simulink model "sampleModel6"  (R2021b)
settings: Solver=VariableStepAuto  StartTime=0.0  StopTime=10.0  RelTol=1e-3
undefined symbols (not defined in the file or in its folder): DiscIntNeverNeededParam
libraries: simulink x11, slpidlib x1
settings Model: Creator=user  LastModifiedBy=user

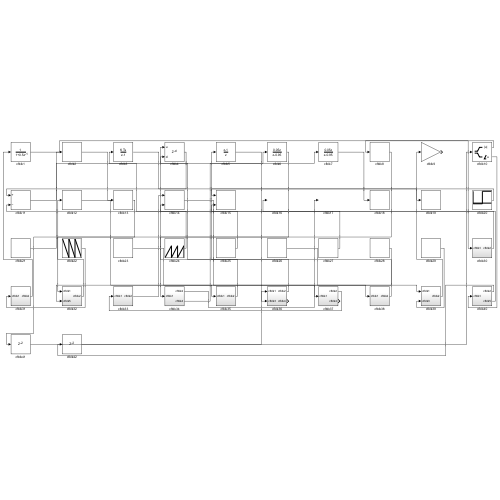
[thumbnail: Simulink's stored preview of the top-level diagram]
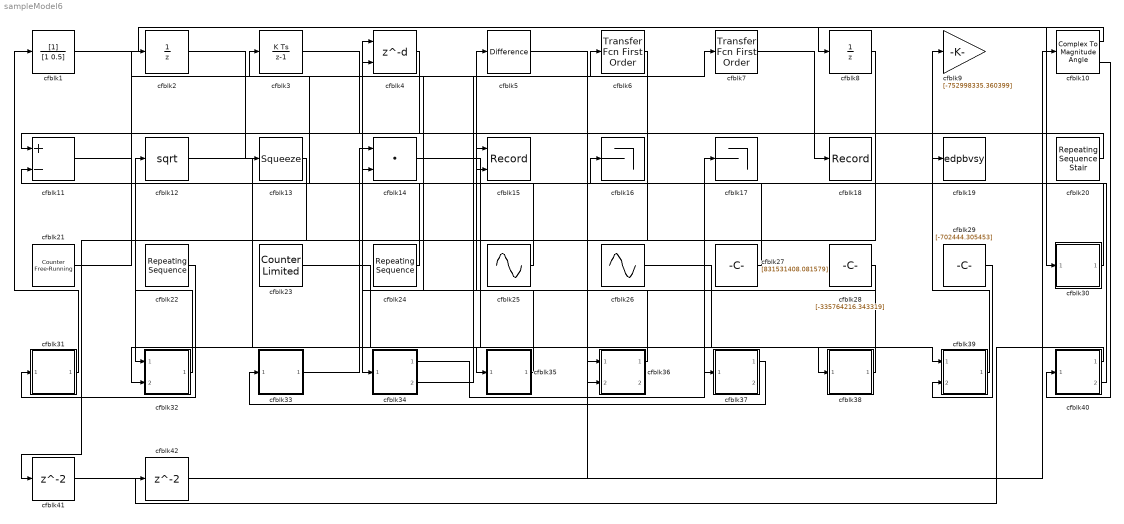
== system sampleModel6 ==
  cfblk1 : DiscreteFilter  SampleTime=1
  cfblk10 : ComplexToMagnitudeAngle
  cfblk11 : Sum  Inputs=+-
  cfblk12 : Sqrt  SaturateOnIntegerOverflow=on
  cfblk13 : Squeeze
  cfblk14 : DotProduct  InputSameDT=on  OutDataTypeStr=Inherit: Inherit via internal rule
  cfblk15 : Record  FileSettingsInternal="{\"entries\":[{\"content\":{\"excelSettings\":{\"content\":{},\"type\":\"Streamout.ExcelSettings\"}},\"type\":\"Streamout.FileSettingStorage\",\"uuid\":\"078a0047-3eb5-4cfb-884a-48a50617e5a1\"}],\"packageUris\":[\"http://schema.mathworks.com/mf0/streamout_blocks/R2020a\"],\"version\":\"1.0\"}"  Layout=[1 1]  SignalsInternal="{\"entries\":[{\"content\":{\"signals\":[{\"content\":{\"blockPath\":[\"sampleModel6/cfblk15\"],\"channel\":[],\"dimensions\":[1],\"domain\":\"sampleModel6/cfblk15\",\"lineColor\":\"#a2142f\",\"plots\":[1],\"port\":1,\"sid\":[\"\"],\"signalID\":237,\"signalName\":\"cfblk20\"},\"type\":\"RecordBlkView.Signal\",\"uuid\":\"e2950a3c-6211-4e69-b9c2-83c3ff1a6d9b\"},{\"content\":{\"blockPath\":[\"sampleModel6/cfblk15\"],\"channel\":[],\"dimensions\":[1],\"domain\":\"sampleModel6/cfblk15\",\"lineColor\":\"#139fff\",\"plots\":[1],\"port\":2,\"sid\":[\"\"],\"signalID\":241,\"signalName\":\"cfblk30\"},\"type\":\"RecordBlkView.Signal\",\"uuid\":\"a62bb186-0eaa-4d5d-9c06-4d8813e13515\"}]},\"type\":\"RecordBlkView.InputSignals\",\"uuid\":\"a1dddcb4-b3bf-44b7-b4b8-68e776bbfcf3\"}],\"packageUris\":[\"http://schema.mathworks.com/mf0/streamout_blocks/R2020a\"],\"version\":\"1.0\"}"  VisualizationBindings="{\"xyplotplugin\":{\"info\":[{\"series\":[{\"bindingParametersList\":[{\"parameter\":\"X-Axis\",\"signalID\":237,\"signalName\":\"cfblk20\"},{\"parameter\":\"Y-Axis\",\"signalID\":241,\"signalName\":\"cfblk30\"}],\"seriesID\":36112}],\"subplotID\":1}]}}"  CompatibilityTag=XY
  cfblk16 : Terminator
  cfblk17 : Terminator
  cfblk18 : Record  FileSettingsInternal="{\"entries\":[{\"content\":{\"excelSettings\":{\"content\":{},\"type\":\"Streamout.ExcelSettings\"}},\"type\":\"Streamout.FileSettingStorage\",\"uuid\":\"ff4303cd-4097-4d51-a6e8-73b3556a0e5d\"}],\"packageUris\":[\"http://schema.mathworks.com/mf0/streamout_blocks/R2020a\"],\"version\":\"1.0\"}"  SignalsInternal="{\"entries\":[{\"content\":{\"signals\":[{\"content\":{\"blockPath\":[\"sampleModel6/cfblk18\"],\"channel\":[],\"dimensions\":[1],\"domain\":\"sampleModel6/cfblk18\",\"lineColor\":\"#d95319\",\"plots\":[1],\"port\":1,\"sid\":[\"\"],\"signalID\":233,\"signalName\":\"cfblk7\"},\"type\":\"RecordBlkView.Signal\",\"uuid\":\"350a4dd6-4f43-4d64-a145-38d7b0e854d1\"}]},\"type\":\"RecordBlkView.InputSignals\",\"uuid\":\"cfb04e90-a252-4558-a39a-d3efc5ac2aac\"}],\"packageUris\":[\"http://schema.mathworks.com/mf0/streamout_blocks/R2020a\"],\"version\":\"1.0\"}"  VisualizationBindings="{\"sparklinesplugin\":{\"info\":[{\"bindingParametersList\":[],\"subplotID\":1}]}}"
  cfblk19 : ToWorkspace  VariableName=edpbvsy  SaveFormat=Timeseries  SampleTime=-1
  cfblk2 : UnitDelay  HasFrameUpgradeWarning=on
  cfblk20 : simulink/Sources/Repeating Sequence Stair  OutValues=[-14722803.076438, 309765796.899337]  tsamp=-1  OutMin=[]  OutMax=[]  OutDataTypeStr=double  OutputDataTypeScalingMode=double  OutDataType=fixdt(0,8)  ConRadixGroup=Best Precision: Vector-wise  OutScaling=2^-12
  cfblk21 : simulink/Sources/Counter Free-Running  NumBits=[53.000000]  tsamp=-1
  cfblk22 : simulink/Sources/Repeating Sequence  rep_seq_t=[0 2]  rep_seq_y=[77051148.938042, -435589670.883555]
  cfblk23 : simulink/Sources/Counter Limited  uplimit=[975.000000]  tsamp=-1
  cfblk24 : simulink/Sources/Repeating Sequence  rep_seq_t=[0 2]  rep_seq_y=[-927148968.949040, -347510853.879375]
  cfblk25 : Sin  Amplitude=[946027247.785641]  Bias=[-269934749.388505]  SampleTime=0
  cfblk26 : Sin  Amplitude=[-381700762.208165]  Bias=[-758175230.838743]  SampleTime=0
  cfblk27 : Constant  Value=[831531408.081579]  SampleTime=1
  cfblk28 : Constant  Value=[-335764216.343319]  SampleTime=1
  cfblk29 : Constant  Value=[-702444.305453]  SampleTime=1
  cfblk3 : DiscreteIntegrator  ICPrevOutput=DiscIntNeverNeededParam  ICPrevScaledInput=DiscIntNeverNeededParam
  cfblk30 : Subsystem
  cfblk31 : Subsystem
  cfblk32 : Subsystem
  cfblk33 : Subsystem
  cfblk34 : Subsystem
  cfblk35 : Subsystem
  cfblk36 : Subsystem
  cfblk37 : Subsystem
  cfblk38 : Subsystem
  cfblk39 : Subsystem
  cfblk4 : Delay  DelayLengthSource=Input port  SampleTime=1
      settings: InputPortMap=u0,p1
  cfblk40 : Subsystem
  cfblk41 : Delay  SampleTime=1
  cfblk42 : Delay  SampleTime=1
  cfblk5 : simulink/Discrete/Difference  ICPrevInput=0.0  OutMin=[]  OutMax=[]  OutDataTypeStr=Inherit: Inherit via back propagation  OutDataType=fixdt(1, 16)  OutScaling=2^-10  DoSatur=off
  cfblk6 : simulink/Discrete/Transfer Fcn First Order  PoleZ=0.95  ICPrevOutput=0.0  DoSatur=off
  cfblk7 : simulink/Discrete/Transfer Fcn First Order  PoleZ=0.95  ICPrevOutput=0.0  DoSatur=off
  cfblk8 : UnitDelay  HasFrameUpgradeWarning=on
  cfblk9 : Gain  Gain=[-752998335.360399]
  wires:
  cfblk12/1 -> cfblk35/1(cfblk1)
  cfblk24/1 -> cfblk3/1
  cfblk32/1(cfblk2) -> cfblk12/1
  cfblk34/1(cfblk2) -> cfblk17/1
  cfblk35/1(cfblk2) -> cfblk5/1
  cfblk1/1 -> cfblk30/1(cfblk1)
  cfblk23/1 -> cfblk38/1(cfblk1)
  cfblk27/1 -> cfblk16/1
  cfblk37/1(cfblk2) -> cfblk33/1(cfblk1)
  cfblk4/1 -> cfblk11/1
  cfblk13/1 -> cfblk32/1(cfblk1)
  cfblk14/1 -> cfblk36/2(cfblk3)
  cfblk8/1 -> cfblk34/1(cfblk1)
  cfblk38/1(cfblk2) -> cfblk4/1
  cfblk31/1(cfblk2) -> cfblk1/1
  cfblk22/1 -> cfblk31/1(cfblk1)
  cfblk25/1 -> cfblk11/2
  cfblk11/1 -> cfblk6/1
  cfblk39/1(cfblk2) -> cfblk9/1
  cfblk10/1 -> cfblk8/1
  cfblk33/1(cfblk2) -> cfblk14/1
  cfblk36/1(cfblk2) -> cfblk4/2
  cfblk21/1 -> cfblk2/1
  cfblk34/2(cfblk4) -> cfblk7/1
  cfblk5/1 -> cfblk37/1(cfblk1)
  cfblk28/1 -> cfblk32/2(cfblk5)
  cfblk26/1 -> cfblk39/1(cfblk1)
  cfblk10/2 -> cfblk40/1(cfblk1)
  cfblk20/1 -> cfblk15/1
  cfblk40/2(cfblk5) -> cfblk14/2
  cfblk7/1 -> cfblk18/1
  cfblk30/1(cfblk2) -> cfblk15/2
  cfblk3/1 -> cfblk19/1
  cfblk29/1 -> cfblk39/2(cfblk3)
  cfblk2/1 -> cfblk13/1
  cfblk6/1 -> cfblk41/1
  cfblk41/1 -> cfblk36/1(cfblk1)
  cfblk40/1(cfblk2) -> cfblk42/1
  cfblk42/1 -> cfblk10/1

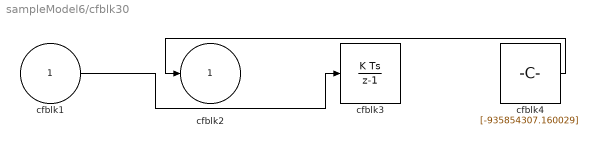
== system sampleModel6/cfblk30 ==
  cfblk1 : Inport
  cfblk3 : DiscreteIntegrator  ICPrevOutput=DiscIntNeverNeededParam  ICPrevScaledInput=DiscIntNeverNeededParam
  cfblk4 : Constant  Value=[-935854307.160029]  SampleTime=1
  cfblk2 : Outport
  wires:
  cfblk4/1 -> cfblk2/1
  cfblk1/1 -> cfblk3/1

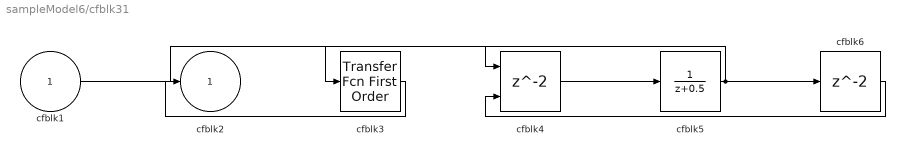
== system sampleModel6/cfblk31 ==
  cfblk1 : Inport
  cfblk3 : simulink/Discrete/Transfer Fcn First Order  PoleZ=0.95  ICPrevOutput=0.0  DoSatur=off
  cfblk4 : Delay  ShowEnablePort=on  SampleTime=1
      settings: InputPortMap=u0,e6
  cfblk5 : DiscreteTransferFcn  SampleTime=1
  cfblk6 : Delay  SampleTime=1
  cfblk2 : Outport
  wires:
  cfblk1/1 -> cfblk4/1
  cfblk3/1 -> cfblk2/1
  cfblk4/1 -> cfblk5/1
  cfblk5/1 -> cfblk3/1, cfblk6/1
  cfblk6/1 -> cfblk4/2

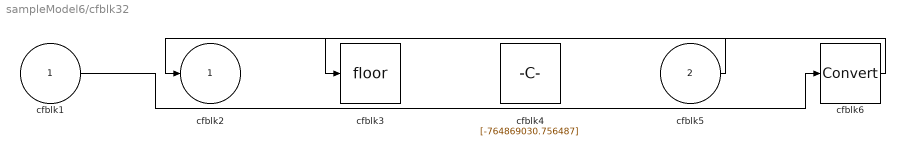
== system sampleModel6/cfblk32 ==
  cfblk1 : Inport
  cfblk5 : Inport  Port=2
  cfblk3 : Rounding
  cfblk4 : Constant  Value=[-764869030.756487]  SampleTime=1
  cfblk6 : DataTypeConversion
  cfblk2 : Outport
  wires:
  cfblk5/1 -> cfblk2/1
  cfblk1/1 -> cfblk6/1
  cfblk6/1 -> cfblk3/1

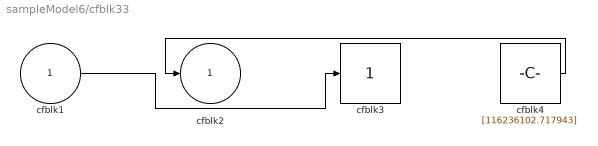
== system sampleModel6/cfblk33 ==
  cfblk1 : Inport
  cfblk3 : simulink/Math Operations/Slider Gain  gain=1  low=0  high=2
  cfblk4 : Constant  Value=[116236102.717943]  SampleTime=1
  cfblk2 : Outport
  wires:
  cfblk4/1 -> cfblk2/1
  cfblk1/1 -> cfblk3/1

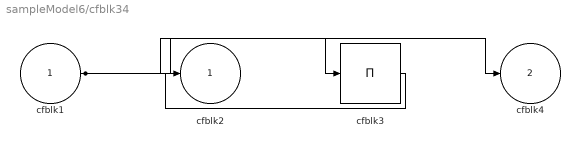
== system sampleModel6/cfblk34 ==
  cfblk1 : Inport
  cfblk3 : Product  Inputs=*
  cfblk2 : Outport
  cfblk4 : Outport  Port=2
  wires:
  cfblk1/1 -> cfblk4/1, cfblk3/1
  cfblk3/1 -> cfblk2/1

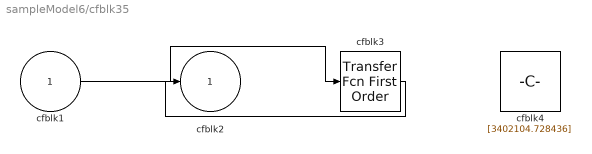
== system sampleModel6/cfblk35 ==
  cfblk1 : Inport
  cfblk3 : simulink/Discrete/Transfer Fcn First Order  PoleZ=0.95  ICPrevOutput=0.0  DoSatur=off
  cfblk4 : Constant  Value=[3402104.728436]  SampleTime=1
  cfblk2 : Outport
  wires:
  cfblk1/1 -> cfblk3/1
  cfblk3/1 -> cfblk2/1

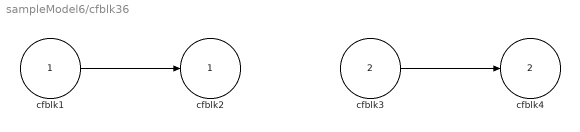
== system sampleModel6/cfblk36 ==
  cfblk1 : Inport
  cfblk3 : Inport  Port=2
  cfblk2 : Outport
  cfblk4 : Outport  Port=2
  wires:
  cfblk1/1 -> cfblk2/1
  cfblk3/1 -> cfblk4/1

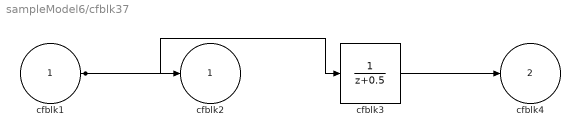
== system sampleModel6/cfblk37 ==
  cfblk1 : Inport
  cfblk3 : DiscreteTransferFcn  SampleTime=1
  cfblk2 : Outport
  cfblk4 : Outport  Port=2
  wires:
  cfblk1/1 -> cfblk2/1, cfblk3/1
  cfblk3/1 -> cfblk4/1

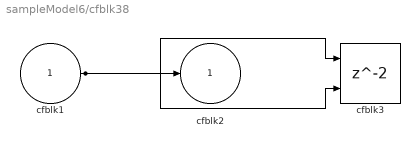
== system sampleModel6/cfblk38 ==
  cfblk1 : Inport
  cfblk3 : Delay  ShowEnablePort=on  SampleTime=1
      settings: InputPortMap=u0,e6
  cfblk2 : Outport
  wires:
  cfblk1/1 -> cfblk2/1, cfblk3/1, cfblk3/2

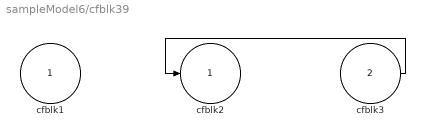
== system sampleModel6/cfblk39 ==
  cfblk1 : Inport
  cfblk3 : Inport  Port=2
  cfblk2 : Outport
  wires:
  cfblk3/1 -> cfblk2/1

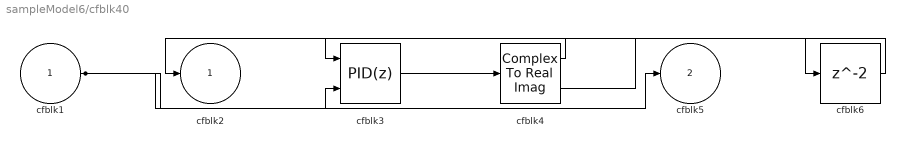
== system sampleModel6/cfblk40 ==
  cfblk1 : Inport
  cfblk3 : slpidlib/PID Controller (2DOF)  Controller=PID  Form=Parallel  TimeDomain=Discrete-time  UseExternalTs=off  SampleTime=1  IntegratorMethod=Forward Euler  FilterMethod=Forward Euler  ControllerParametersSource=internal  P=1  I=1  D=0  UseFilter=on  N=100  b=1  c=1  TunerSelectOption=Transfer Function Based (PID Tuner App)  InitialConditionSource=internal  InitialConditionForIntegrator=0  InitialConditionForFilter=0  DifferentiatorICPrevScaledInput=0  ExternalReset=none  TrackingMode=off  Kt=1  LimitOutput=off  SatLimitsSource=internal  UpperSaturationLimit=inf  LowerSaturationLimit=-inf  LinearizeAsGain=off  AntiWindupMode=none  Kb=1  POutMin=[]  POutMax=[]  IOutMin=[]  IOutMax=[]  DOutMin=[]  DOutMax=[]  NOutMin=[]  NOutMax=[]  bOutMin=[]  bOutMax=[]  cOutMin=[]  cOutMax=[]  SumOutMin=[]  SumOutMax=[]  SaturationOutMin=[]  SaturationOutMax=[]  PParamMin=[]  PParamMax=[]  IParamMin=[]  IParamMax=[]  DParamMin=[]  DParamMax=[]  NParamMin=[]  NParamMax=[]  bParamMin=[]  bParamMax=[]  cParamMin=[]  cParamMax=[]  KbParamMin=[]  KbParamMax=[]  KtParamMin=[]  KtParamMax=[]  KbOutMin=[]  KbOutMax=[]  KtOutMin=[]  KtOutMax=[]  IntegratorOutMin=[]  IntegratorOutMax=[]  FilterOutMin=[]  FilterOutMax=[]  SumI1OutMin=[]  SumI1OutMax=[]  SumI2OutMin=[]  SumI2OutMax=[]  SumI3OutMin=[]  SumI3OutMax=[]  SumI4OutMin=[]  SumI4OutMax=[]  SumDOutMin=[]  SumDOutMax=[]  Sum1OutMin=[]  Sum1OutMax=[]  Sum2OutMin=[]  Sum2OutMax=[]  Sum3OutMin=[]  Sum3OutMax=[]  DifferentiatorOutMin=[]  DifferentiatorOutMax=[]  FilterDiffOutCoefMin=[]  FilterDiffOutCoefMax=[]  ReciprocalOutMin=[]  ReciprocalOutMax=[]  SumDenOutMin=[]  SumDenOutMax=[]  SumNumOutMin=[]  SumNumOutMax=[]  DivideOutMin=[]  DivideOutMax=[]  UdiffTsProdOutMin=[]  UdiffTsProdOutMax=[]  NTsProdOutMin=[]  NTsProdOutMax=[]  UintegralTsProdOutMin=[]  UintegralTsProdOutMax=[]  UngainTsProdOutMin=[]  UngainTsProdOutMax=[]  IntegratorContinuousStateAttributes=''  IntegratorStateMustResolveToSignalObject=off  IntegratorRTWStateStorageClass=Auto  FilterContinuousStateAttributes=''  FilterStateMustResolveToSignalObject=off  FilterRTWStateStorageClass=Auto  ParallelPVariant=InternalParameters  IdealPVariant=Disabled  IVariant=InternalParameters  DVariant=InternalParameters  bVariant=InternalParameters  cVariant=InternalParameters  IntegratorVariant=Discrete  SatVariant=Disabled  AWVariant=Passthrough  PCopyVariant=Disabled  TRVariant=Disabled  FdbkBlocksVariant=Forward  IdealPFdbkVariant=Disabled  SatFdbkVariant=Disabled  DerivativeFilterVariant=ForwardEulerFilter  NVariant=InternalParameters  NCopyVariant=Disabled  FilterICVariant=InternalICsFilter  IntegratorICVariant=InternalICs  ExternalResetVariant=Disabled  TRSumVariant=Passthrough  SumFdbkVariant=Disabled  SumVariant=Sum_PID  TsampFilterVariant=InternalTs  TsampNgainVariant=Passthrough  TsampIntegralVariant=Passthrough  ExternalSaturationOutDataTypeStr=Inherit: Same as second input
      settings: SourceProductBaseCode=SL
  cfblk4 : ComplexToRealImag
  cfblk6 : Delay  SampleTime=1
  cfblk2 : Outport
  cfblk5 : Outport  Port=2
  wires:
  cfblk3/1 -> cfblk4/1
  cfblk4/1 -> cfblk2/1
  cfblk1/1 -> cfblk5/1, cfblk3/2
  cfblk4/2 -> cfblk6/1
  cfblk6/1 -> cfblk3/1
